simulink library "csu_rfm_rate_fusion_model_lib"  (R2014b)
settings: Solver=ode45  SolverMode=SingleTasking  StartTime=0.0  StopTime=10.0  RelTol=1e-3
values from neighbouring files (symbols this model uses):
  sim_time_step_size = 0.01    [csu_lak_linear_accel_kinematics_test.m]
undefined symbols (not defined in the file or in its folder): gyk_miru_gyro_dcm_in_chu
libraries: util_info_lib x1, util_quat_lib x1, util_common_lib x1
settings Model: Creator=hcannon  LastModifiedBy=mstewart

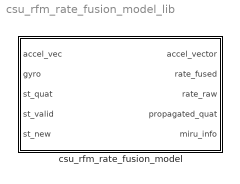
== system csu_rfm_rate_fusion_model_lib ==
  csu_rfm_rate_fusion_model : Subsystem

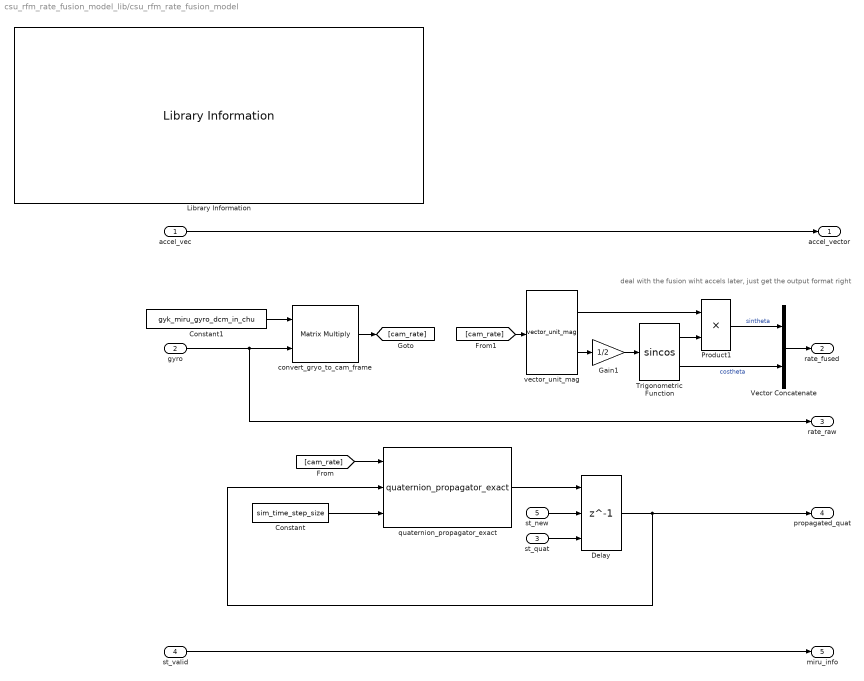
== system csu_rfm_rate_fusion_model_lib/csu_rfm_rate_fusion_model ==
  note: deal with the fusion wiht accels later, just get the output format right
  accel_vec : Inport
  gyro : Inport  Port=2
  st_quat : Inport  Port=3
  st_valid : Inport  Port=4
  st_new : Inport  Port=5
  Constant : Constant  Value=sim_time_step_size  OutDataTypeStr=double
  Constant1 : Constant  Value=gyk_miru_gyro_dcm_in_chu  OutDataTypeStr=double
  Delay : Delay  DelayLength=1  InitialConditionSource=Input port  InitialCondition=0  ExternalReset=Rising
      settings: InputPortMap=u0,r5,p4
  Gain1 : Gain  Gain=1/2
  Library Information : util_info_lib/Library Information  owner='escrane'
  Product1 : Product  RndMeth=Zero
  Trigonometric Function : Trigonometry  Operator=sincos
  Vector Concatenate : Concatenate
  convert_gryo_to_cam_frame : Product  Multiplication=Matrix(*)  RndMeth=Zero
  quaternion_propagator_exact : util_quat_lib/quaternion_propagator_exact  SystemSampleTime=-1
  vector_unit_mag : util_common_lib/vector_unit_mag  SystemSampleTime=-1
  accel_vector : Outport
  rate_fused : Outport  Port=2
  rate_raw : Outport  Port=3
  propagated_quat : Outport  Port=4
  miru_info : Outport  Port=5
  wires:
  accel_vec/1 -> accel_vector/1
  gyro/1 -> rate_raw/1, convert_gryo_to_cam_frame/2
  st_valid/1 -> miru_info/1
  Constant/1 -> quaternion_propagator_exact/3
  quaternion_propagator_exact/1 -> Delay/1
  Delay/1 -> quaternion_propagator_exact/2, propagated_quat/1
  st_quat/1 -> Delay/3
  st_new/1 -> Delay/2
  Constant1/1 -> convert_gryo_to_cam_frame/1
  convert_gryo_to_cam_frame/1 -> [cam_rate]
  [cam_rate] -> quaternion_propagator_exact/1
  Gain1/1 -> Trigonometric Function/1
  Product1/1 -> Vector Concatenate/1  "sintheta"
  vector_unit_mag/1 -> Product1/1
  Trigonometric Function/2 -> Vector Concatenate/2  "costheta"
  Trigonometric Function/1 -> Product1/2
  Vector Concatenate/1 -> rate_fused/1
  vector_unit_mag/2 -> Gain1/1
  [cam_rate] -> vector_unit_mag/1
